simulink model "PIDCodigo_Punto_3C"  (R2023b)
settings: Solver=VariableStepAuto  StartTime=0.0  StopTime=10.0  RelTol=1e-3
settings Model: Creator=juanvillegas  LastModifiedBy=juanr

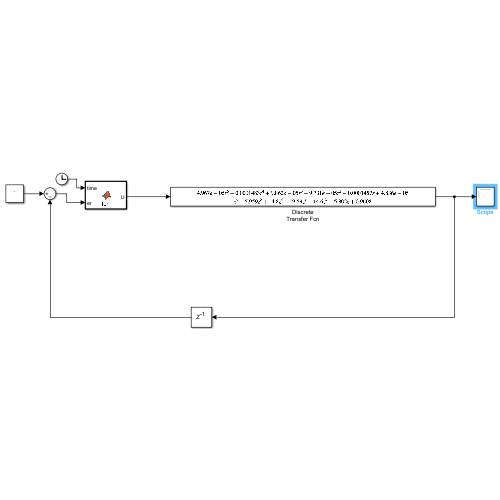
[thumbnail: Simulink's stored preview of the top-level diagram]
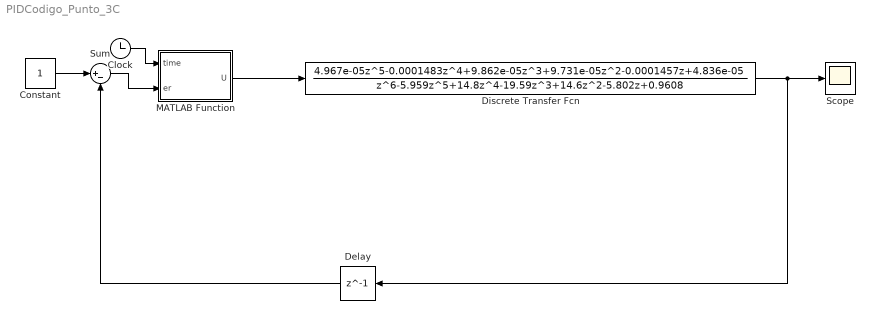
== system PIDCodigo_Punto_3C ==
  Clock : Clock
  Constant : Constant
  Delay : Delay  DelayLength=1
  Discrete Transfer Fcn : DiscreteTransferFcn  Numerator=[4.967e-05, -0.0001483, 9.862e-05, 9.731e-05, -0.0001457, 4.836e-05]  Denominator=[1, -5.959, 14.8, -19.59, 14.6, -5.802, 0.9608]
  MATLAB Function : MATLAB Function  TreatAsAtomicUnit=on
  Scope : Scope
  Sum : Sum  Inputs=|+-
  wires:
  Clock/1 -> MATLAB Function/1(time)
  Constant/1 -> Sum/1
  Sum/1 -> MATLAB Function/2(er)
  Delay/1 -> Sum/2
  MATLAB Function/1(U) -> Discrete Transfer Fcn/1
  Discrete Transfer Fcn/1 -> Delay/1, Scope/1

== matlab function PIDCodigo_Punto_3C/MATLAB Function ==
  data: time input; U output; er input
function U = fcn(time,er)

persistent erm1 erm2 dm1 dm2 d1 T_ant
Ts=0.02;
consKp_1=180;
consKi_1=89;
consKd_1=90.8;
%%consKd_1=0;
if(isempty(erm1))
    erm1=0;
    erm2=0;
    dm1=0;
    dm2=0;
    d1=0;
    T_ant=0;
else 
  erm2=erm1;
  erm1=er;
  dm2=dm1;
  dm1=d1;
end

if (time-T_ant>Ts)
  
  T_ant=time;
  K1=consKp_1+(consKi_1*Ts/2)+(consKd_1*2/Ts);
  K2=(consKi_1*Ts)-(consKd_1*4/Ts);
  K3=(consKi_1*Ts/2)-consKp_1+(consKd_1*2/Ts);
  d1=er*K1+erm1*K2+erm2*K3+dm2;


    if(d1>250)
        d1=250;
    end

    if(d1<10)
        d1=10;
    end
end 

U=d1;
